simulink subsystem "P2D_ROM"  (R2022a)
settings: Solver=VariableStepAuto  StartTime=0.0  StopTime=10.0  RelTol=1e-3
values from neighbouring files (symbols this model uses):
  Ts = sim_data.impl.SIM.Ts    [P2D_System_main.m]    (also in P2D_System_main_sine.m; runSimulink.m = sim_in.SIM.Ts)
  x0_ROM = zeros(length(A_r),1)    [P2D_System_main.m]    (also in P2D_System_main_sine.m; runSimulink.m = Slink.x0_ROM)
undefined symbols (not defined in the file or in its folder): A_ROM, B_ROM, C_ROM
settings Model: Creator=tyevans  LastModifiedBy=tyevans

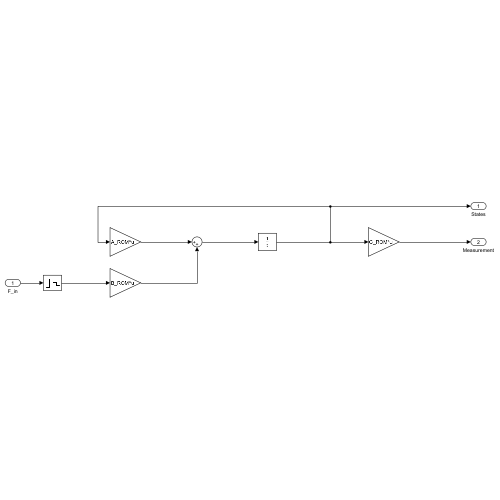
[thumbnail: Simulink's stored preview of the top-level diagram]
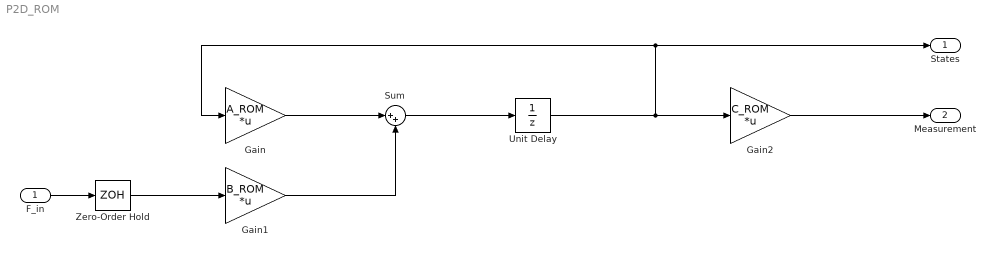
== system P2D_ROM ==
  F_in : Inport
  Gain : Gain  Gain=A_ROM  Multiplication=Matrix(K*u)
  Gain1 : Gain  Gain=B_ROM  Multiplication=Matrix(K*u)
  Gain2 : Gain  Gain=C_ROM  Multiplication=Matrix(K*u)
  Sum : Sum  Inputs=|++
  Unit Delay : UnitDelay  InitialCondition=x0_ROM  SampleTime=-1  HasFrameUpgradeWarning=on
  Zero-Order Hold : ZeroOrderHold  SampleTime=Ts
  States : Outport
  Measurement : Outport  Port=2
  wires:
  Unit Delay/1 -> Gain2/1, Gain/1, States/1
  Gain2/1 -> Measurement/1
  F_in/1 -> Zero-Order Hold/1
  Gain/1 -> Sum/1
  Sum/1 -> Unit Delay/1
  Gain1/1 -> Sum/2
  Zero-Order Hold/1 -> Gain1/1
